simulink model "EcoSIM3_P2_C2_WIP"  (R2014b)
settings: Solver=ode1  SolverMode=SingleTasking  StartTime=0.0  StopTime=4  FixedStep=0.01  RelTol=1e-3
PostLoadFcn:
  | %, if any(exist('dsrtsu_mdlpostloadfcn', 'file') == [2, 3, 6]), try dsrtsu_mdlpostloadfcn('Execute', bdroot); catch fprintf('Error in PostLoadFcn (dsrtsu_mdlpostloadfcn) for model "%s":\n %s\n', bdroot, lasterr); end, end,
InitFcn:
  | tic
  | %Startup_EcoSIM
undefined symbols (not defined in the file or in its folder): canChannel, Controls, DriveCycles, Driver, EM_EFF_MAP, EM_PwrLoss_MAP, EngPwr, EngSpd, EngTrq, Glbl, Overwritten_Mode, Plants, Power, sigbuilder_block, Torque, Trialmap, Veh_Dynamics
libraries: simulink x135, canmsglib x113, fl_lib x104, canlib x89, nesl_utility x56, sdl_lib x29, dspsigops x6, dspswit3 x5, dspstat3 x2, commnoisgen2 x1, dspfdesign x1
(part 21 of 21)

== stateflow chart EcoSIM3_P2_C2_WIP/Supervisory Controller/Mode Selection /Start-Stop control/Engine_Start_Stop ==
  state Engine_Start
    en, du: Mode = 4;
    Time_in_wait = 0;
  state Engine_Only
    en, du: Mode = 3;
    Time_in_wait = 0;
  state Engine_Wait_State
    en, du: Mode = 3;
    Time_in_wait = 1;
  state Engine_Stop
    en, du: Mode = 2;
    Time_in_wait = 0;
  (default) -> (junction 38)
  Engine_Stop -> Engine_Start : [Alpha_Percent>2]
  (junction 38) -> Engine_Start [order 2]
  (junction 38) -> Engine_Only [order 1] : [eng_running==1]
  Engine_Start -> Engine_Only : [eng_running==1]
  Engine_Only -> Engine_Wait_State : [Alpha_Percent==0 &&...
      | Vehicle_Speed<=1]
  Engine_Wait_State -> Engine_Only [order 1] : [Alpha_Percent>0&&...
      | Time_to_Stop<Time_in_wait_limit]
  Engine_Wait_State -> Engine_Stop [order 2] : [Time_to_Stop>Time_in_wait_limit]
  data: Vehicle_Speed input; Brake_Pedal_Position input; Alpha_Percent input; eng_running input; Mode output; Time_in_wait output; Time_in_wait_limit input; Time_to_Stop input

== stateflow chart EcoSIM3_P2_C2_WIP/Supervisory Controller/Mode Operation/Engine Only /Trans Clutch Messages/AggressiveClutchRelease ==
  state Entry
    entry: Shift_Request=0;
  state EngagementTransition
    entry: Shift_Request=0;
    exit: Shift_Request=0;
    state LowSpeed
      entry: Shift_Request=0;
    state Transition
      entry: Shift_Request=0.5*(BAS_Speed-Lower_Clutch_Speed);
      during: Shift_Request=0.5*(BAS_Speed-Lower_Clutch_Speed);
    state FullyEngaged
      entry: Shift_Request=100;
    (default) -> LowSpeed
    Transition -> LowSpeed [order 1] : [BAS_Speed<=Lower_Clutch_Speed]
    FullyEngaged -> LowSpeed [order 1] : [BAS_Speed<=Lower_Clutch_Speed]
    LowSpeed -> Transition : [BAS_Speed>185+5]
    Transition -> FullyEngaged [order 2] : [BAS_Speed>=375+5]
    FullyEngaged -> Transition [order 2] : [BAS_Speed<Upper_Clutch_Speed]
  (default) -> Entry
  EngagementTransition -> Entry : [Clutch_Request==0]
  Entry -> EngagementTransition : [Clutch_Request==1]
  data: BAS_Speed input; Clutch_Request input; Lower_Clutch_Speed input; Upper_Clutch_Speed input; Shift_Request output

== stateflow chart EcoSIM3_P2_C2_WIP/Powertrain/Accessories Power Module/Subsystem/Algorithm/CAN fault ==
  state Normal
    entry:
    CANdown=0;
    count=0;
    state=1;
  state Abnormal
    entry:
    count=1;
    state=2;
    during:
    count=count+1;
  state Fault
    entry:
    CANdown=1;
    state=0;
  (default) -> Normal
  Normal -> Abnormal : [LowVoltEnblRq ~=0 && LowVoltEnblRq ~=1 && PowerUp>0]
  Fault -> Normal : [PowerUp==0]
  Abnormal -> Normal [order 2] : [LowVoltEnblRq ==0 || LowVoltEnblRq ==1]
  Abnormal -> Fault [order 1] : [count>=10]
  data: CANdown output; PowerUp input; LowVoltEnblRq input; count local; state output

== stateflow chart EcoSIM3_P2_C2_WIP/Powertrain/Accessories Power Module/Subsystem/Algorithm/DC-DC SoftECU ==
  state Working
    state Enable
      entry:
      AccPwrMdlLowVlt=0;
      AccPwrMdlLwVltSysFld=0;
      State=2;
      during:
    state Operation
      entry:
      AccPwrMdlLowVlt=LwVltStpntCmnd;
      AccPwrMdlLwVltSysFld=0;
      State=3;
      during:
      AccPwrMdlLowVlt=LwVltStpntCmnd;
    (default) -> Enable
    Operation -> Enable : [LowVoltEnblRq==0]
    Enable -> Operation : [LowVoltEnblRq==1]
  state Off
    entry:
    AccPwrMdlLowVlt=0;
    AccPwrMdlLwVltSysFld=0;
    State=1;
  state Fault
    entry:
    AccPwrMdlLowVlt=0;
    AccPwrMdlLwVltSysFld=1;
    State=0;
    during:
  Working -> Fault [order 1] : [Fault==1 || CANdown==1]
  Off -> Working [order 2] : [PowerUp>0  && bcm_mainc_stat==1]
  Working -> Off [order 2] : [PowerUp==0  || bcm_mainc_stat==0]
  (default) -> Off
  Off -> Fault [order 1] : [Fault==1]
  Fault -> Off : [Fault==0 && PowerUp==0]
  data: CANdown input; State output; PowerUp input; LowVoltEnblRq input; bcm_mainc_stat input; LwVltStpntCmnd input; Fault input boolean; bcmVbat input; PowerReq input; AccPwrMdlLowVlt output; AccPwrMdlLwVltSysFld output

== stateflow chart EcoSIM3_P2_C2_WIP/Powertrain/Accessories Power Module/Plant/Chart ==
  state Inactive
    entry:
    APMLwVltOtptCrntUns=0;
    AccPwrMdlHiVltInpCrnt=0;
  state Active
    entry:
    APMLwVltOtptCrntUns=PowerReq/AccPwrMdlLowVlt;
    AccPwrMdlHiVltInpCrnt=PowerReq/bcmVbat/.98;
    during:
    APMLwVltOtptCrntUns=PowerReq/AccPwrMdlLowVlt;
    AccPwrMdlHiVltInpCrnt=PowerReq/bcmVbat/.98;
  (default) -> Inactive
  Inactive -> Active : [AccPwrMdlLowVlt~=0]
  data: APMLwVltOtptCrntUns output; AccPwrMdlHiVltInpCrnt output; AccPwrMdlLowVlt input; PowerReq input; bcmVbat input
